simulink model "sedemo_arq_gobackn"  (Simulink 7.5)
settings: Solver=VariableStepDiscrete  StartTime=0.0  StopTime=50  MaxStep=inf  RelTol=1e-3
PreLoadFcn:
  | SWS=7;
  | Tframe=0.1;
  | Tprop = 1;
  | Pe = 0.1;
PostLoadFcn:
  | sedemo_arq_gobackn_settings;
libraries: simeventsserver1 x7, simeventssink1 x6, simeventsattributes2 x5, simeventstranslate1 x4, simeventsrouting1 x4, simeventsgenerators1 x3, simeventsqueue1 x2, simeventsgates1 x2, simeventsprobes1 x1, simeventsinfo x1, simeventssignalmanage1 x1
CloseFcn:
  | clear arq;
  | clear Pe;
  | clear SWS;
  | clear Tframe;
  | clear Tprop;
settings Model: Creator=The MathWorks Inc.  ExtModeAutoUpdateStatusClock=off
settings SolverCC: InsertRTBMode=Auto
settings DataIOCC: SaveOutput=off  SaveTime=off
settings OptimizationCC: InitFltsAndDblsToZero=on
settings DebuggingCC: AlgebraicLoopMsg=error  SignalResolutionControl=TryResolveAllWithWarning  SolverPrmCheckMsg=none  MultiTaskDSMMsg=warning  MultiTaskCondExecSysMsg=none  StrictBusMsg=Warning
settings RTWCC: IncludeERTFirstTime=on
settings SimEventsCC: propDiagAttribOutput=1  propDiagFcnCallOutput=0  propDiagStatOutput=0

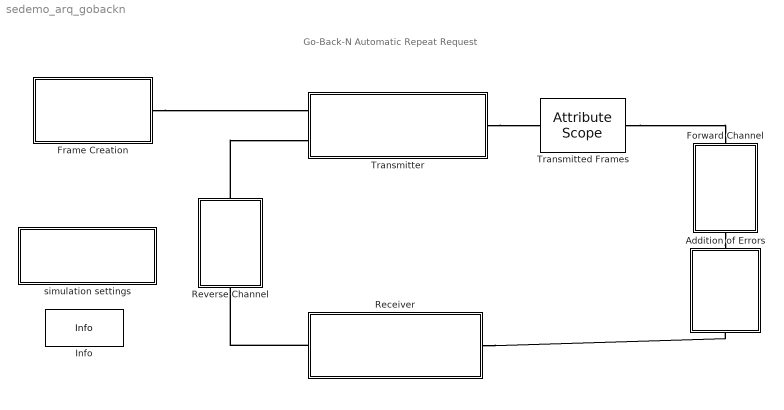
== system sedemo_arq_gobackn ==
  note: Go-Back-N Automatic Repeat Request
  Addition of Errors : Subsystem
  Forward Channel : Subsystem
  Frame Creation : Subsystem
  Info : simeventsinfo/Info  SystemSampleTime=-1
  Receiver : Subsystem
  Reverse Channel : Subsystem
  Transmitted Frames : simeventssink1/Attribute Scope  Priority=1  SystemSampleTime=-1  PlotType=Stem  InputType=Attribute  NumInputs=1  AttributeNameY=seqNum  XInputOptionSignal=Event time  XInputOptionEntity=Event time  AttributeNameX=Count  EnableEntityOutport=on  XMin=-0.494689305558682  XMax=49.9636198614269  XLimitExceededOption=Stretch axis limits  YLimitExceededOption=Stretch axis limits  AxisGrid=on  AxisLegend=off  LineDisables=""  LineColors=b  LineStyles=-  LineMarkers=.  OpenScopeAtSimStart=on  Title=Transmitted Frames  YLabel=Sequence Number  XLabel=Time  FigurePosition=[34 295 257 200]  AxisZoom=off  DataStoreOption=Limited  DataPointsLimit=10000  StatNumberArrived=Off  ShowCountPlotted=off  ShowToolbar=off
      settings: YMin=-0.57  YMax=57.57
  Transmitter : Subsystem
  simulation settings : Subsystem  mask(simulation settings){SWS=7, Tframe=.1, Tprop=1, Pe=.1}
      mask prompts: SWS "Sliding window size:"; Tframe "Time to transmit frame:"; Tprop "Propagation time:"; Pe "Probability of erroneous frame:"
      mask help:
      | Parameter settings for Go-Back-N Automatic Repeat Request (ARQ) model.
      |
      | Sliding window size: Maximum number of unacknowledged frames allowed in transit at any time
      |
      | Time to transmit frame: Amount of time it takes transmitter to send out all bits in a given frame
      |
      | Propagation time: Amount of time for a frame to propagate one way from the transmitter to the receiver or vice versa.  This should be longer than the time to transmit a frame.
      |
      | Probability of erroneous frame: Probability that a frame will be corrupted in transit, requiring it to be resent
      mask init:
      | sedemo_arq_gobackn_settings;
      mask Help: eval('simeventsdemohelp')
      mask Display: disp('Double-click to change\nsimulation settings')
  connections:
  Transmitter/RConn1 -- Transmitted Frames/LConn1
  Forward Channel/RConn1 -- Addition of Errors/LConn1
  Transmitted Frames/RConn1 -- Forward Channel/LConn1
  Receiver/LConn1 -- Addition of Errors/RConn1
  Receiver/RConn1 -- Reverse Channel/LConn1
  Reverse Channel/RConn1 -- Transmitter/LConn2
  Frame Creation/RConn1 -- Transmitter/LConn1

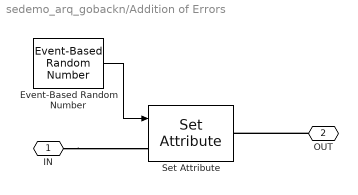
== system sedemo_arq_gobackn/Addition of Errors ==
  Event-Based Random Number : simeventsgenerators1/Signal Generators/Event-Based Random Number  SystemSampleTime=-1  distribution=Bernoulli  meanExp=1  minUnif=0  maxUnif=1  pOneBern=1-Pe  pSuccessBino=0.5  numTrialBino=1  meanNorm=0  stdNorm=1  minTri=1  maxTri=3  modeTri=2  thresholdLogn=0  scaleLogn=1  shapeLogn=1  pSuccessGeo=0.5  meanPoiss=1  thresholdLogl=0  scaleLogl=1  thresholdGam=0  scaleGam=1  shapeGam=1  minBeta=0  maxBeta=1  shape1Beta=1  shape2Beta=1  minUnid=0  maxUnid=1  numValueUnid=2  thresholdWbl=0  scaleWbl=1  shapeWbl=1  valueVecCont=[0 1]  cdfVecCont=[0 1]  valueVecDisc=[0 1]  probVecDisc=[0.5 0.5]  seed=12345  IsProcessed=on  isConnected=1
  Set Attribute : simeventsattributes2/Set Attribute  Priority=1  DialogController=des_ddg_create  DialogControllerArgs=DataTag1  SystemSampleTime=-1  AttributeFrom=Signal port  AttributeName=crc_check  AttributeTreatAsVector=1  AttributeValue=0  AttributeCreate=on  StatNumberDeparted=Off  EvaluatedAttributeValue={[]}
  IN : PMIOPort  Port=1  Side=Left
  OUT : PMIOPort  Port=2  Side=Right
  wires:
  Event-Based Random Number/1 -> Set Attribute/1
  connections:
  OUT/RConn1 -- Set Attribute/RConn1
  IN/RConn1 -- Set Attribute/LConn1

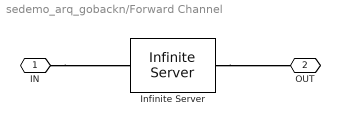
== system sedemo_arq_gobackn/Forward Channel ==
  Infinite Server : simeventsserver1/Infinite Server  Priority=1  SystemSampleTime=-1  ServiceTimeFrom=Dialog  ServiceTime=Tprop  AttributeName=ServiceTime  PriorityServiceCompletion=500  EnableTOPort=off  StatNumberDeparted=Off  StatNumberInBlock=Off  StatPendingEntity=Off  StatNumberPending=Off  StatAverageWait=Off  StatNumberTimedout=Off
  IN : PMIOPort  Port=1  Side=Left
  OUT : PMIOPort  Port=2  Side=Right
  connections:
  IN/RConn1 -- Infinite Server/LConn1
  Infinite Server/RConn1 -- OUT/RConn1

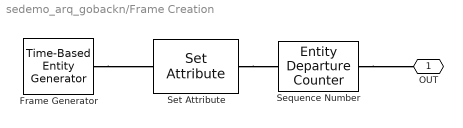
== system sedemo_arq_gobackn/Frame Creation ==
  Frame Generator : simeventsgenerators1/Entity Generators/Time-Based Entity Generator  Priority=1  DialogController=des_ddg_create  DialogControllerArgs=DataTag4  SystemSampleTime=-1  GenerateEntitiesUpon=Intergeneration time from dialog  Distribution=Exponential  Minimum=0  Maximum=3  Mean=1  InitialSeed=2367  Period=1  PriorityEntityGeneration=1000  GenerateEntityAtSimulationStart=on  ResponseWhenBlocked=Pause generation  ResponseWhenUnblocked=Immediate restart  EntityType=Blank  StatNumberDeparted=Off  StatPendingEntity=Off  StatAverageIntergenerationTime=Off
  Sequence Number : simeventsprobes1/Entity Departure Counter  Priority=1  SystemSampleTime=-1  NumberDepartedToSignal=Off  NumberDepartedToAttribute=On  NumberDepartedAttributeName=seqNum  CreateAttribute=on  CounterResetTypeOption=Off  CounterResetEdgeOption=Rising  SpecifyEventPriority=off  PriorityEntityCounterReset=1
  Set Attribute : simeventsattributes2/Set Attribute  Priority=1  DialogController=des_ddg_create  DialogControllerArgs=DataTag7  SystemSampleTime=-1  AttributeFrom=Dialog  AttributeName=seqNum  AttributeTreatAsVector=1  AttributeValue=0  AttributeCreate=on  StatNumberDeparted=Off  EvaluatedAttributeValue={0}
  OUT : PMIOPort  Port=1  Side=Right
  connections:
  Sequence Number/RConn1 -- OUT/RConn1
  Frame Generator/RConn1 -- Set Attribute/LConn1
  Set Attribute/RConn1 -- Sequence Number/LConn1

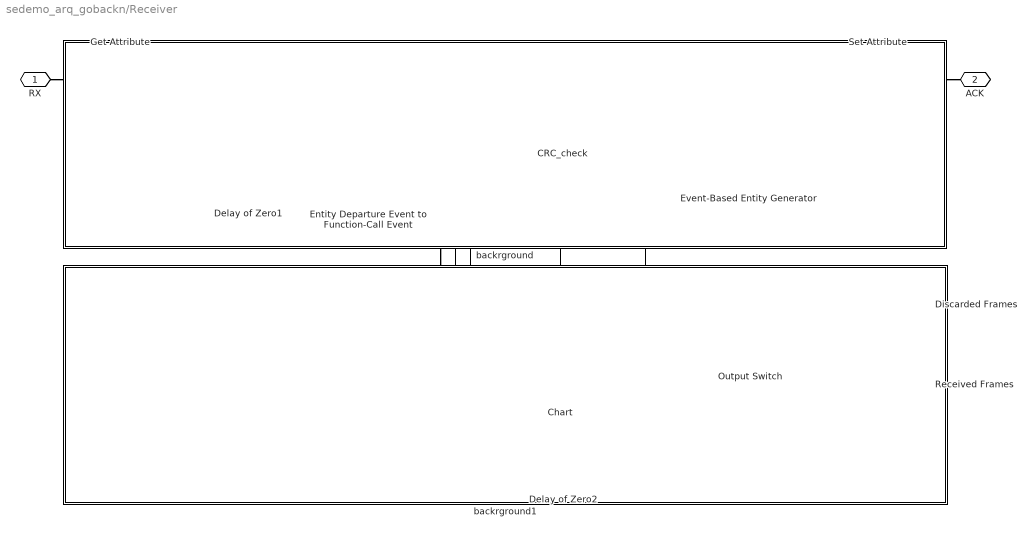
== system sedemo_arq_gobackn/Receiver ==
  CRC_check : simeventssink1/Signal Scope  Priority=1  SystemSampleTime=-1  PlotType=Stair  InputType=Signal  NumInputs=1  AttributeNameY=Count  XInputOptionSignal=Event time  XInputOptionEntity=Event time  AttributeNameX=Count  EnableEntityOutport=on  XMin=-0.494296279481752  XMax=49.923924227657  XLimitExceededOption=Stretch axis limits  YLimitExceededOption=Stretch axis limits  AxisGrid=on  AxisLegend=off  LineDisables=""  LineColors=b  LineStyles=-  LineMarkers=.  OpenScopeAtSimStart=on  Title=CRC Check  YLabel=""  XLabel=Time  FigurePosition=[300 542 267 171]  AxisZoom=off  DataStoreOption=Limited  DataPointsLimit=10000  StatNumberArrived=Off  ShowCountPlotted=off  ShowToolbar=off
      settings: YMin=-0.01  YMax=1.01
  Chart : Stateflow chart  TreatAsAtomicUnit=on
      settings: PropExecContextOutsideSubsystem=on
  Delay of Zero1 : simeventsserver1/Infinite Server  Priority=1  SystemSampleTime=-1  ServiceTimeFrom=Dialog  ServiceTime=0  AttributeName=ServiceTime  PriorityServiceCompletion=10  EnableTOPort=off  StatNumberDeparted=Off  StatNumberInBlock=Off  StatPendingEntity=Off  StatNumberPending=Off  StatAverageWait=Off  StatNumberTimedout=Off
  Delay of Zero2 : simeventsserver1/Infinite Server  Priority=1  SystemSampleTime=-1  ServiceTimeFrom=Dialog  ServiceTime=0  AttributeName=ServiceTime  PriorityServiceCompletion=10  EnableTOPort=off  StatNumberDeparted=Off  StatNumberInBlock=Off  StatPendingEntity=Off  StatNumberPending=Off  StatAverageWait=Off  StatNumberTimedout=Off
  Discarded Frames : simeventssink1/Attribute Scope  Priority=1  SystemSampleTime=-1  PlotType=Stem  InputType=Attribute  NumInputs=1  AttributeNameY=seqNum  XInputOptionSignal=Event time  XInputOptionEntity=Event time  AttributeNameX=Count  EnableEntityOutport=off  XMin=-0.476542207053357  XMax=48.1307629123891  XLimitExceededOption=Stretch axis limits  YLimitExceededOption=Stretch axis limits  AxisGrid=on  AxisLegend=off  LineDisables=""  LineColors=b  LineStyles=-  LineMarkers=.  OpenScopeAtSimStart=on  Title=Discarded Frames  YLabel=Sequence Number  XLabel=Time  FigurePosition=[299 295 269 199]  AxisZoom=off  DataStoreOption=Limited  DataPointsLimit=10000  StatNumberArrived=Off  ShowCountPlotted=off  ShowToolbar=off
      settings: YMin=-0.53  YMax=53.53
  Entity Departure Event to Function-Call Event : simeventstranslate1/Entity Departure Event to Function-Call Event  Priority=1  SystemSampleTime=-1  TimingFunctionCallF1=After entity departure  EnableE1Port=off  EnableF2Port=off  TimingFunctionCallF2=Before entity departure  EnableE2Port=off  StatNumberDeparted=Off  StatNumberF1Calls=Off  StatNumberF2Calls=Off  IsInsideAFB=off
  Event-Based Entity Generator : simeventsgenerators1/Entity Generators/Event-Based Entity Generator  Priority=1  DialogController=des_ddg_create  DialogControllerArgs=DataTag14  SystemSampleTime=-1  GenerateEntitiesUpon=Function call from port fcn  SignalEdgeType=Rising  SpecifyEventPriority=on  PriorityEntityGeneration=1  GenerateEntityAtSimulationStart=off  AllowBlocking=off  ResponseDuringBlockage=Discard generated entities  EntityType=Blank  StatNumberDeparted=Off  StatPendingEntity=Off  StatAverageIntergenerationTime=Off
  Get Attribute : simeventsattributes2/Get Attribute  Priority=1  DialogController=des_ddg_create  DialogControllerArgs=DataTag16  SystemSampleTime=-1  AttributeName=crc_check|seqNum  AttributeMissing=Error|Error  AttributeDefaultValue=0|0  AttributeSendTiming=After entity departure|After entity departure  AttributeTreatAsVector=1|1  StatNumberDeparted=Off  EvaluatedDefaultAttributeValue={[];[]}
  Output Switch : simeventsrouting1/Output Switch  Priority=1  SystemSampleTime=-1  NumberOutputPorts=2  SwitchingCriterion=From signal port p  InitialSeed=34567  AttributeName=Attribute1  InitialConditionsOpt=off  InitialConditions=1  EntityBufferOpt=off  SpecifyEventPriority=off  PriorityOutputSwitchSelectPort=4100  TimeoutPortOpt=off  StatNumberDeparted=Off  StatNumberTimedOut=Off  StatPendingEntity=Off  StatLastDeparturePort=Off  EvaluatedNumPorts=2
  Received Frames : simeventssink1/Attribute Scope  Priority=1  SystemSampleTime=-1  PlotType=Stem  InputType=Attribute  NumInputs=1  AttributeNameY=seqNum  XInputOptionSignal=Event time  XInputOptionEntity=Event time  AttributeNameX=Count  EnableEntityOutport=off  XMin=-0.494296279481752  XMax=49.923924227657  XLimitExceededOption=Stretch axis limits  YLimitExceededOption=Stretch axis limits  AxisGrid=on  AxisLegend=off  LineDisables=""  LineColors=b  LineStyles=-  LineMarkers=.  OpenScopeAtSimStart=on  Title=Received Frames  YLabel=Sequence Number  XLabel=Time  FigurePosition=[576 295 271 199]  AxisZoom=off  DataStoreOption=Limited  DataPointsLimit=10000  StatNumberArrived=Off  ShowCountPlotted=off  ShowToolbar=off
      settings: YMin=-0.55  YMax=55.55
  Set Attribute : simeventsattributes2/Set Attribute  Priority=1  DialogController=des_ddg_create  DialogControllerArgs=DataTag20  SystemSampleTime=-1  AttributeFrom=Signal port|Signal port  AttributeName=ack|seqNum  AttributeTreatAsVector=1|1  AttributeValue=0|0  AttributeCreate=on  StatNumberDeparted=Off  EvaluatedAttributeValue={[];[]}
  backrground : Subsystem
      mask Display: disp('')
  backrground1 : Subsystem
      mask Display: disp('')
  RX : PMIOPort  Port=1  Side=Left
  ACK : PMIOPort  Port=2  Side=Right
  wires:
  Get Attribute/1 -> Set Attribute/1, Chart/1(crc_check), CRC_check/1
  Get Attribute/2 -> Set Attribute/2, Chart/2(seqNum)
  Entity Departure Event to Function-Call Event/1 -> Chart/Trigger
  Chart/2(send_ack) -> Event-Based Entity Generator/1
  Chart/1(p) -> Output Switch/1
  connections:
  RX/RConn1 -- Get Attribute/LConn1
  Get Attribute/RConn1 -- Delay of Zero1/LConn1
  Delay of Zero1/RConn1 -- Entity Departure Event to Function-Call Event/LConn1
  Event-Based Entity Generator/RConn1 -- Set Attribute/LConn1
  Set Attribute/RConn1 -- ACK/RConn1
  Discarded Frames/LConn1 -- Output Switch/RConn1
  Received Frames/LConn1 -- Output Switch/RConn2
  Entity Departure Event to Function-Call Event/RConn1 -- Delay of Zero2/LConn1
  Delay of Zero2/RConn1 -- Output Switch/LConn1

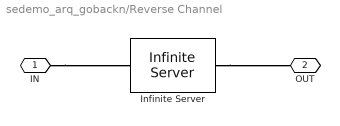
== system sedemo_arq_gobackn/Reverse Channel ==
  Infinite Server : simeventsserver1/Infinite Server  Priority=1  SystemSampleTime=-1  ServiceTimeFrom=Dialog  ServiceTime=Tprop  AttributeName=ServiceTime  PriorityServiceCompletion=501  EnableTOPort=off  StatNumberDeparted=Off  StatNumberInBlock=Off  StatPendingEntity=Off  StatNumberPending=Off  StatAverageWait=Off  StatNumberTimedout=Off
  IN : PMIOPort  Port=1  Side=Left
  OUT : PMIOPort  Port=2  Side=Right
  connections:
  Infinite Server/RConn1 -- OUT/RConn1
  IN/RConn1 -- Infinite Server/LConn1

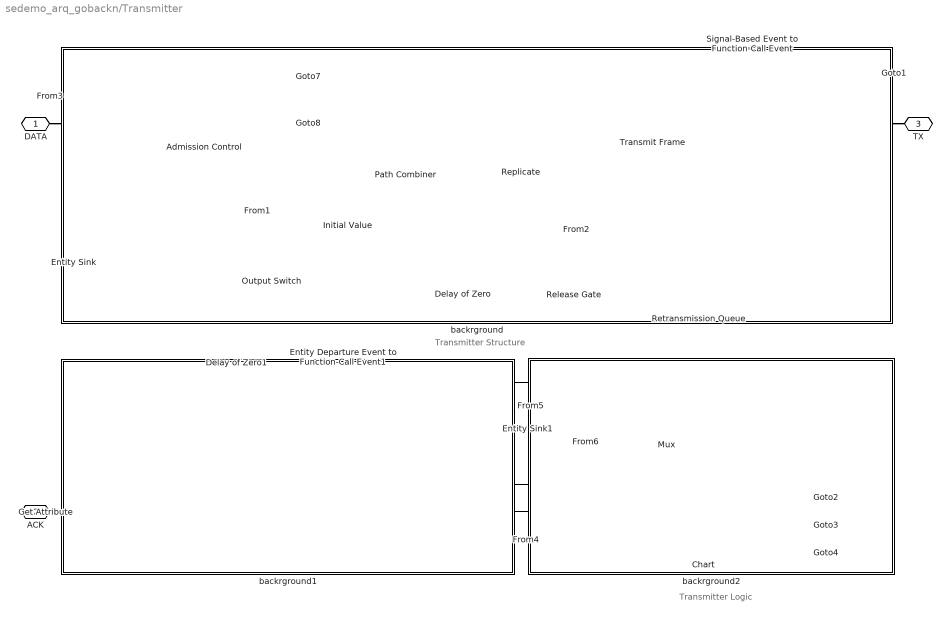
== system sedemo_arq_gobackn/Transmitter ==
  note: Transmitter Structure
  note: Transmitter Logic
  Admission Control : Subsystem
  Chart : Stateflow chart  TreatAsAtomicUnit=on
      settings: PropExecContextOutsideSubsystem=on
  Delay of Zero : simeventsserver1/Infinite Server  Priority=1  SystemSampleTime=-1  ServiceTimeFrom=Dialog  ServiceTime=0  AttributeName=ServiceTime  PriorityServiceCompletion=10  EnableTOPort=off  StatNumberDeparted=Off  StatNumberInBlock=Off  StatPendingEntity=Off  StatNumberPending=Off  StatAverageWait=Off  StatNumberTimedout=Off
  Delay of Zero1 : simeventsserver1/Infinite Server  Priority=1  SystemSampleTime=-1  ServiceTimeFrom=Dialog  ServiceTime=0  AttributeName=ServiceTime  PriorityServiceCompletion=10  EnableTOPort=off  StatNumberDeparted=Off  StatNumberInBlock=Off  StatPendingEntity=Off  StatNumberPending=Off  StatAverageWait=Off  StatNumberTimedout=Off
  Entity Departure Event to Function-Call Event1 : simeventstranslate1/Entity Departure Event to Function-Call Event  Priority=1  SystemSampleTime=-1  TimingFunctionCallF1=After entity departure  EnableE1Port=off  EnableF2Port=off  TimingFunctionCallF2=Before entity departure  EnableE2Port=off  StatNumberDeparted=Off  StatNumberF1Calls=Off  StatNumberF2Calls=Off  IsInsideAFB=off
  Entity Sink : simeventssink1/Entity Sink  Priority=1  SystemSampleTime=-1  AvailableForArrivals=on  StatNumberArrived=Off
  Entity Sink1 : simeventssink1/Entity Sink  Priority=1  SystemSampleTime=-1  AvailableForArrivals=on  StatNumberArrived=Off
  Get Attribute : simeventsattributes2/Get Attribute  Priority=1  DialogController=des_ddg_create  DialogControllerArgs=DataTag32  SystemSampleTime=-1  AttributeName=ack|seqNum  AttributeMissing=Error|Error  AttributeDefaultValue=0|0  AttributeSendTiming=After entity departure|After entity departure  AttributeTreatAsVector=1|1  StatNumberDeparted=Off  EvaluatedDefaultAttributeValue={[];[]}
  Initial Value : simeventssignalmanage1/Initial Value  InitialValue=2
  Mux : Mux  Inputs=3
  Output Switch : simeventsrouting1/Output Switch  Priority=1  SystemSampleTime=-1  NumberOutputPorts=2  SwitchingCriterion=From signal port p  InitialSeed=34567  AttributeName=Attribute1  InitialConditionsOpt=off  InitialConditions=1  EntityBufferOpt=off  SpecifyEventPriority=off  PriorityOutputSwitchSelectPort=1  TimeoutPortOpt=off  StatNumberDeparted=Off  StatNumberTimedOut=Off  StatPendingEntity=Off  StatLastDeparturePort=Off  EvaluatedNumPorts=2
  Path Combiner : simeventsrouting1/Path Combiner  Priority=1  SystemSampleTime=-1  NumberInputPorts=2  InputPortPrecedence=IN1 port  InitialSeed=45675  SpecifyEventPriority=off  PriorityPathCombinerPortPrecedenceSelection=4100  StatNumberDeparted=Off  StatLastArrivalPort=Off  EvaluatedNumPorts=2
  Release Gate : simeventsgates1/Release Gate  Priority=1  SystemSampleTime=-1  OpenGateUpon=Function call from port fcn  SignalEdgeOption=Rising  SpecifyEventPriority=off  PriorityGateRelease=2  StatNumberDeparted=Off
  Replicate : simeventsrouting1/Replicate  Priority=1  SystemSampleTime=-1  NumberOutputPorts=2  ReplicateEntityWhen=All entity output ports are not blocked  OutputPortPrecedence=OUT1 port  InitialSeed=56789  ActionUponBlocking=Discard entity  StatNumberArrived=Off  StatNumberDeparted=Off  EvaluatedNumPorts=2
  Retransmission Queue : simeventsqueue1/FIFO Queue  Priority=1  SystemSampleTime=-1  Capacity=SWS  EnableTOPort=off  StatNumberDeparted=Off  StatNumberInBlock=Off  StatPendingEntity=Off  StatAverageWait=Off  StatAverageQueueLength=Off  StatNumberTimedout=Off
  Signal-Based Event to Function-Call Event : simeventstranslate1/Signal-Based Event to Function-Call Event  Priority=1  SystemSampleTime=-1  GenerateFunctionCallUpon=Change in signal from port vc  SignalEdgeOption=Falling  EnableE1Port=off  EnableF2Port=off  EnableE2Port=off  SpecifyEventPriority=on  PriorityFunctionCall=200  FunctionCallDelayFrom=Dialog  DelayFunctionCall=0  StatNumberF1Calls=Off  StatNumberF2Calls=Off  MaskBlockType=none
  Transmit Frame : simeventsserver1/Single Server  Priority=1  SystemSampleTime=-1  ServiceTimeFrom=Dialog  ServiceTime=Tframe  AttributeName=ServiceTime  PriorityServiceCompletion=100  PermitPreemption=off  SortingAttributeName=PriorityAttributeName  SortingDirection=Ascending  WriteToAttribute=off  ResidualAttributeName=ResidualServiceTime  CreateAttribute=on  EnableTOPort=off  StatNumberDeparted=Off  StatNumberInBlock=On  StatNumberPreempted=Off  StatPendingEntity=Off  StatAverageWait=Off  StatUtilization=Off  StatNumberTimedout=Off
  backrground : Subsystem
      mask Display: disp('')
  backrground1 : Subsystem
      mask Display: disp('')
  backrground2 : Subsystem
      mask Display: disp('')
  DATA : PMIOPort  Port=1  Side=Left
  ACK : PMIOPort  Port=2  Side=Left
  TX : PMIOPort  Port=3  Side=Right
  wires:
  Mux/1 -> Chart/Trigger
  [tx] -> Admission Control/1(tx)
  Admission Control/2(frameReady) -> [frameReady]
  Admission Control/1(new_frame) -> [new_frame]
  [retx] -> Release Gate/1
  Entity Departure Event to Function-Call Event1/1 -> Mux/1
  Get Attribute/1 -> Chart/1(ack)
  Get Attribute/2 -> Chart/2(seqNum)
  [frameReady] -> Chart/3(frameReady)
  Chart/1(p) -> [p]
  Chart/2(tx) -> [tx]
  Chart/3(retx) -> [retx]
  [new_frame] -> Mux/2
  [link_open] -> Mux/3
  Transmit Frame/1 -> Signal-Based Event to Function-Call Event/1
  Signal-Based Event to Function-Call Event/1 -> [link_open]
  Initial Value/1 -> Output Switch/1
  [p] -> Initial Value/1
  connections:
  Delay of Zero1/RConn1 -- Entity Departure Event to Function-Call Event1/LConn1
  Entity Departure Event to Function-Call Event1/RConn1 -- Entity Sink1/LConn1
  ACK/RConn1 -- Get Attribute/LConn1
  Get Attribute/RConn1 -- Delay of Zero1/LConn1
  Path Combiner/RConn1 -- Replicate/LConn1
  Retransmission Queue/RConn1 -- Release Gate/LConn1
  Delay of Zero/LConn1 -- Release Gate/RConn1
  Replicate/RConn2 -- Retransmission Queue/LConn1
  Transmit Frame/RConn1 -- TX/RConn1
  DATA/RConn1 -- Admission Control/LConn1
  Admission Control/RConn1 -- Path Combiner/LConn1
  Replicate/RConn1 -- Transmit Frame/LConn1
  Output Switch/RConn1 -- Path Combiner/LConn2
  Output Switch/LConn1 -- Delay of Zero/RConn1
  Entity Sink/LConn1 -- Output Switch/RConn2

== system sedemo_arq_gobackn/simulation settings ==

== system sedemo_arq_gobackn/Receiver/backrground ==

== system sedemo_arq_gobackn/Receiver/backrground1 ==

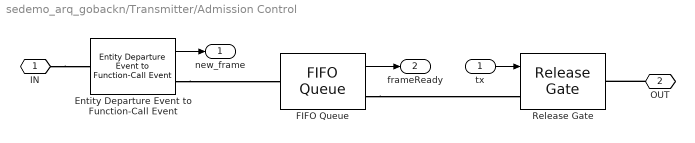
== system sedemo_arq_gobackn/Transmitter/Admission Control ==
  tx : Inport  OutDataType=sfix(16)  OutScaling=2^0
  Entity Departure Event to Function-Call Event : simeventstranslate1/Entity Departure Event to Function-Call Event  Priority=1  SystemSampleTime=-1  TimingFunctionCallF1=After entity departure  EnableE1Port=off  EnableF2Port=off  TimingFunctionCallF2=Before entity departure  EnableE2Port=off  StatNumberDeparted=Off  StatNumberF1Calls=Off  StatNumberF2Calls=Off  IsInsideAFB=off
  FIFO Queue : simeventsqueue1/FIFO Queue  Priority=1  SystemSampleTime=-1  Capacity=1  EnableTOPort=off  StatNumberDeparted=Off  StatNumberInBlock=On  StatPendingEntity=Off  StatAverageWait=Off  StatAverageQueueLength=Off  StatNumberTimedout=Off
  Release Gate : simeventsgates1/Release Gate  Priority=1  SystemSampleTime=-1  OpenGateUpon=Function call from port fcn  SignalEdgeOption=Rising  SpecifyEventPriority=off  PriorityGateRelease=2200  StatNumberDeparted=Off
  IN : PMIOPort  Port=1  Side=Left
  OUT : PMIOPort  Port=2  Side=Right
  new_frame : Outport  OutDataType=sfix(16)  OutScaling=2^0
  frameReady : Outport  Port=2  OutDataType=sfix(16)  OutScaling=2^0
  wires:
  Entity Departure Event to Function-Call Event/1 -> new_frame/1
  tx/1 -> Release Gate/1
  FIFO Queue/1 -> frameReady/1
  connections:
  Entity Departure Event to Function-Call Event/RConn1 -- FIFO Queue/LConn1
  FIFO Queue/RConn1 -- Release Gate/LConn1
  IN/RConn1 -- Entity Departure Event to Function-Call Event/LConn1
  OUT/RConn1 -- Release Gate/RConn1

== system sedemo_arq_gobackn/Transmitter/backrground ==

== system sedemo_arq_gobackn/Transmitter/backrground1 ==

== system sedemo_arq_gobackn/Transmitter/backrground2 ==

== stateflow chart Transmitter/Chart ==
  state Transmitting
    % Placing a new data frame on the link
    en: LFS++; tx;
    on new_ack: p=2; retx; LAR=seqNum; % Positive ACK
  state Retransmitting
    % Retransmitting data frames across link
    en: p=1; retx; retxCount=LFS-LAR-1;
    on link_open: retx; retxCount--;
  state Idle
    % Not transmitting because no new data
    % is available or the maximum number of
    % outstanding frames has been reached
  state WaitingToRetransmit
    % Waiting for link to become available in order
    % to start retransmission of rejected frames
  (default) -> Transmitting : {LAR=0; LFS=0;p=1;}
  Transmitting -> (junction 7) [order 2] : link_open
  (junction 7) -> Idle [order 1] : [frameReady==0 | LFS-LAR==SWS]
  (junction 7) -> Transmitting [order 2]
  Idle -> Retransmitting [order 2] : new_ack [ack==0]
      | % Negative ACK
  Transmitting -> WaitingToRetransmit [order 1] : new_ack [ack==0]
      | % Negative ACK
  WaitingToRetransmit -> Retransmitting : link_open
  Retransmitting -> (junction 7) : link_open [retxCount==0]
      | % Finished retransmitting
  Idle -> (junction 7) [order 1] : new_ack [ack==1]
      | {p=2; retx; LAR=seqNum;}
      | % Positive ACK
  Idle -> (junction 7) [order 3] : new_frame
  data: ack input double; p output double; seqNum input double; LAR local double; retxCount local double; SWS parameter double =3; LFS local double; frameReady input double
  events: tx output FUNCTION_CALL_EVENT; retx output FUNCTION_CALL_EVENT; new_ack input FUNCTION_CALL_EVENT; new_frame input FUNCTION_CALL_EVENT; link_open input FUNCTION_CALL_EVENT

== stateflow chart Receiver/Chart ==
  state Accepting
    % Accept incoming frames until
    % a corrupted frame is received
    en: p=2; LFR=seqNum; send_ack;
  state Waiting
    % Disregard incoming frames until the
    % next frame in sequence is received.
    en: p=1; send_ack;
  (default) -> (junction 35)
  (junction 35) -> Accepting [order 1] : [crc_check==1]
  (junction 35) -> Waiting [order 2]
  Accepting -> (junction 35)
  Waiting -> (junction 35) : [seqNum==LFR+1]
  data: crc_check input double; p output double; LFR local double; seqNum input double
  events: new_frame input FUNCTION_CALL_EVENT; send_ack output FUNCTION_CALL_EVENT
